simulink model "PID_Test"  (R2023b)
settings: Solver=VariableStepAuto  StartTime=0.0  StopTime=50  MaxStep=1  RelTol=1e-3  AbsTol=1e-3
InitFcn:
  | addpath('Schwungmasse/Schwungmasse_Matlab/Schwungmassenmodell_softHIL')
  | addpath('../');
  | 
  | if exist('systunePIDd', 'var')
  |     disp('systunePID exists!');
  | else
  |     MotorMitSchwungmasseTuner; % tune PID using systune
  | end
  | 
  | if ~exist('geneticPIDd', 'var') | ~exist('differentialPIDd', 'var')
  |     GeneticAndDifferentialParams; % init genetic and differential PIDs
  | end
undefined symbols (not defined in the file or in its folder): differentialPIDd, geneticPIDd, getservername, systunePIDd
libraries: slpidlib x3, simulink x2
settings Model: Creator=mkottman  LastModifiedBy=Alex
settings SolverCC: AutoScaleAbsTol=off  AlgebraicLoopSolver=TrustRegion
settings DataIOCC: SaveFormat=Array  SignalLoggingSaveFormat=ModelDataLogs  SaveOutput=off  SaveTime=off  ReturnWorkspaceOutputs=off
settings OptimizationCC: BooleanDataType=off  ExpressionDepthLimit=2147483647  InitFltsAndDblsToZero=on  LifeSpan=inf
settings DebuggingCC: SaveWithParameterizedLinksMsg=none  UnderspecifiedInitializationDetection=Classic  MergeDetectMultiDrivingBlocksExec=none  SignalResolutionControl=TryResolveAllWithWarning  MultiTaskDSMMsg=warning  MultiTaskCondExecSysMsg=none  FcnCallInpInsideContextMsg=warning  UnconnectedInputMsg=warning  UnconnectedOutputMsg=warning  UnconnectedLineMsg=warning  StateNameClashWarn=warning  SFUnexpectedBacktrackingDiag=warning  SFNoUnconditionalDefaultTransitionDiag=warning  SFExecutionAtInitializationDiag=none  ArithmeticOperatorsInVariantConditions=warning
settings HardwareCC: ProdBitPerPointer=32  ProdBitPerSizeT=32  ProdBitPerPtrDiffT=32  ProdLargestAtomicFloat=None  ProdIntDivRoundTo=Undefined  ProdEndianess=Unspecified  ProdWordSize=32  ProdHWDeviceType=32-bit Generic  TargetUnknown=on
settings ModelReferenceCC: EnableRefExpFcnMdlSchedulingChecks=on  PropagateSignalLabelsOutOfModel=off
settings SFSimCC: SimUseLocalCustomCode=off  CustomCodeUndefinedFunction=UseInterfaceOnly
settings RTWCC: TemplateMakefile=grt_vc.tmf  RTWUseLocalCustomCode=off
settings CodeAppCC: StateflowObjectComments=on
settings GRTTargetCC: TargetFcnLib=ansi_tfl_tmw.mat  TargetLangStandard=C89/C90 (ANSI)  CombineOutputUpdateFcns=off  GRTInterface=on
settings ConfigComp: CovMetricSettings=dw  CovSaveCumulativeToWorkspaceVar=on  CovSaveSingleToWorkspaceVar=on  CovExternalEMLEnable=off

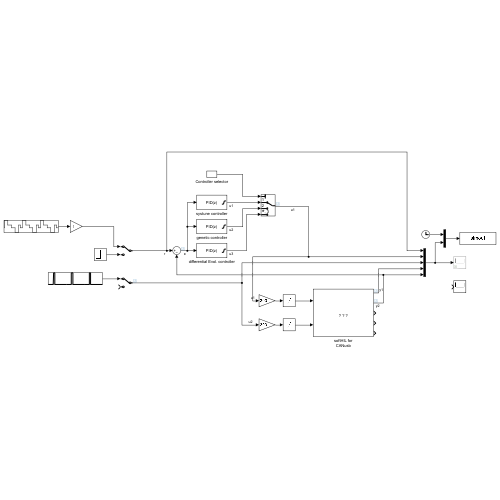
[thumbnail: Simulink's stored preview of the top-level diagram]
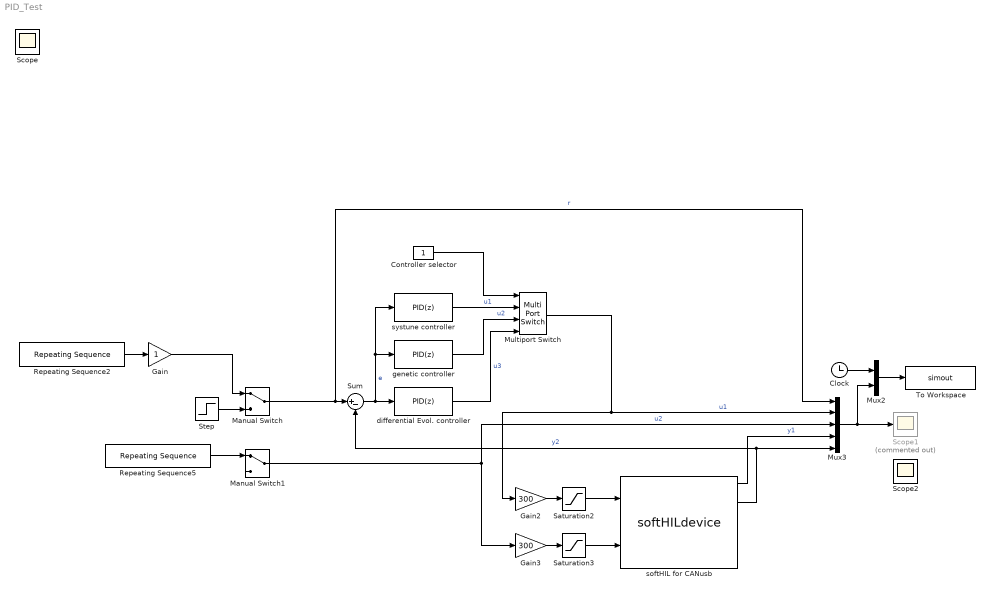
== system PID_Test ==
  Clock : Clock
  Controller selector : Constant
  Gain : Gain
  Gain2 : Gain  Gain=300
  Gain3 : Gain  Gain=300
  Manual Switch : ManualSwitch
  Manual Switch1 : ManualSwitch
  Multiport Switch : MultiPortSwitch  SaturateOnIntegerOverflow=off  InputSameDT=off
  Mux2 : Mux  Inputs=2
  Mux3 : Mux  Inputs=5
  Repeating Sequence2 : simulink/Sources/Repeating Sequence  rep_seq_t=[0.000000 0.490000 0.500000 9.990000 10.000000 19.990000 20.000000 29.990000 30.000000 39.990000 40.000000 44.990000 45.000000 49.990000 50.000000 ]  rep_seq_y=[0.000000 0.000000 31.415927 31.415927 12.566371 12.566371 0.000000 0.000000 -18.849556 -18.849556 12.566371 12.566371 0.000000 0.000000 0.000000 ]
  Repeating Sequence5 : simulink/Sources/Repeating Sequence  rep_seq_t=[0.000000 13.990000 14.000000 17.990000 18.000000 49.990000 50.000000 ]  rep_seq_y=[0.000000 0.000000 10.000000 10.000000 0.000000 0.000000 0.000000 ]
  Saturation2 : Saturate  UpperLimit=3000  LowerLimit=-3000
  Saturation3 : Saturate  UpperLimit=3000  LowerLimit=-3000
  Scope1 : Scope  Commented=on
  Scope2 : Scope
  Step : Step  Time=5  After=3.14159265/2  SampleTime=0.01
  Sum : Sum  Inputs=|+-
  To Workspace : ToWorkspace  VariableName=simout  SampleTime=0.01
  differential Evol. controller : slpidlib/PID Controller  Controller=PID  Form=Parallel  TimeDomain=Discrete-time  UseExternalTs=off  SampleTime=0.01  IntegratorMethod=Forward Euler  FilterMethod=Forward Euler  ControllerParametersSource=internal  P=differentialPIDd.Kp  I=differentialPIDd.Ki  UseKiTs=off  D=differentialPIDd.Kd  N=1/differentialPIDd.Tf  UseFilter=on  TunerSelectOption=Transfer Function Based (PID Tuner App)  InitialConditionSource=internal  InitialConditionForIntegrator=0  InitialConditionForFilter=0  DifferentiatorICPrevScaledInput=0  ExternalReset=none  TrackingMode=off  Kt=1  LimitOutput=on  SatLimitsSource=internal  UpperSaturationLimit=10  LowerSaturationLimit=-10  LinearizeAsGain=on  AntiWindupMode=clamping  Kb=1  LimitIntegrator=off  UpperIntegratorSaturationLimit=10  LowerIntegratorSaturationLimit=-10  POutMin=[]  POutMax=[]  IOutMin=[]  IOutMax=[]  DOutMin=[]  DOutMax=[]  NOutMin=[]  NOutMax=[]  SumOutMin=[]  SumOutMax=[]  SaturationOutMin=[]  SaturationOutMax=[]  PParamMin=[]  PParamMax=[]  IParamMin=[]  IParamMax=[]  DParamMin=[]  DParamMax=[]  NParamMin=[]  NParamMax=[]  KbParamMin=[]  KbParamMax=[]  KtParamMin=[]  KtParamMax=[]  KbOutMin=[]  KbOutMax=[]  KtOutMin=[]  KtOutMax=[]  IntegratorOutMin=[]  IntegratorOutMax=[]  FilterOutMin=[]  FilterOutMax=[]  SumI1OutMin=[]  SumI1OutMax=[]  SumI2OutMin=[]  SumI2OutMax=[]  SumI3OutMin=[]  SumI3OutMax=[]  SumI4OutMin=[]  SumI4OutMax=[]  SumDOutMin=[]  SumDOutMax=[]  DifferentiatorOutMin=[]  DifferentiatorOutMax=[]  FilterDiffOutCoefMin=[]  FilterDiffOutCoefMax=[]  ReciprocalOutMin=[]  ReciprocalOutMax=[]  SumDenOutMin=[]  SumDenOutMax=[]  SumNumOutMin=[]  SumNumOutMax=[]  DivideOutMin=[]  DivideOutMax=[]  UdiffTsProdOutMin=[]  UdiffTsProdOutMax=[]  NTsProdOutMin=[]  NTsProdOutMax=[]  UintegralTsProdOutMin=[]  UintegralTsProdOutMax=[]  UngainTsProdOutMin=[]  UngainTsProdOutMax=[]  ClampingZeroOutDataTypeStr=Inherit: Inherit via back propagation  ClampingZeroOutMin=[]  ClampingZeroOutMax=[]  FilterDenConstantOutDataTypeStr=Inherit: Inherit via back propagation  FilterDenConstantOutMin=[]  FilterDenConstantOutMax=[]  PCopyOutDataTypeStr=Inherit: Inherit via back propagation  PCopyOutMin=[]  PCopyOutMax=[]  NCopyOutDataTypeStr=Inherit: Inherit via back propagation  NCopyOutMin=[]  NCopyOutMax=[]  IntegratorContinuousStateAttributes=''  IntegratorStateMustResolveToSignalObject=off  IntegratorRTWStateStorageClass=Auto  FilterContinuousStateAttributes=''  FilterStateMustResolveToSignalObject=off  FilterRTWStateStorageClass=Auto  ParallelPVariant=InternalParameters  IdealPVariant=Disabled  IVariant=InternalParameters  DVariant=InternalParameters  IntegratorVariant=Discrete  SatVariant=Enabled  AWVariant=DiscClampingParallel  PCopyVariant=Disabled  TRVariant=Disabled  FdbkBlocksVariant=Forward  IdealPFdbkVariant=Disabled  SatFdbkVariant=Disabled  DerivativeFilterVariant=ForwardEulerFilter  NVariant=InternalParameters  NCopyVariant=Disabled  FilterICVariant=InternalICsFilter  IntegratorICVariant=InternalICs  ExternalResetVariant=Disabled  TRSumVariant=Passthrough  SumFdbkVariant=Disabled  SumVariant=Sum_PID  TsampFilterVariant=InternalTs  TsampNgainVariant=Passthrough  TsampIntegralVariant=Disabled_SignalSpec  ExternalSaturationOutDataTypeStr=Inherit: Same as second input
  genetic controller : slpidlib/PID Controller  Controller=PID  Form=Parallel  TimeDomain=Discrete-time  UseExternalTs=off  SampleTime=0.01  IntegratorMethod=Forward Euler  FilterMethod=Forward Euler  ControllerParametersSource=internal  P=geneticPIDd.Kp  I=geneticPIDd.Ki  UseKiTs=off  D=geneticPIDd.Kd  N=1/geneticPIDd.Tf  UseFilter=on  TunerSelectOption=Transfer Function Based (PID Tuner App)  InitialConditionSource=internal  InitialConditionForIntegrator=0  InitialConditionForFilter=0  DifferentiatorICPrevScaledInput=0  ExternalReset=none  TrackingMode=off  Kt=1  LimitOutput=on  SatLimitsSource=internal  UpperSaturationLimit=10  LowerSaturationLimit=-10  LinearizeAsGain=on  AntiWindupMode=clamping  Kb=1  LimitIntegrator=off  UpperIntegratorSaturationLimit=10  LowerIntegratorSaturationLimit=-10  POutMin=[]  POutMax=[]  IOutMin=[]  IOutMax=[]  DOutMin=[]  DOutMax=[]  NOutMin=[]  NOutMax=[]  SumOutMin=[]  SumOutMax=[]  SaturationOutMin=[]  SaturationOutMax=[]  PParamMin=[]  PParamMax=[]  IParamMin=[]  IParamMax=[]  DParamMin=[]  DParamMax=[]  NParamMin=[]  NParamMax=[]  KbParamMin=[]  KbParamMax=[]  KtParamMin=[]  KtParamMax=[]  KbOutMin=[]  KbOutMax=[]  KtOutMin=[]  KtOutMax=[]  IntegratorOutMin=[]  IntegratorOutMax=[]  FilterOutMin=[]  FilterOutMax=[]  SumI1OutMin=[]  SumI1OutMax=[]  SumI2OutMin=[]  SumI2OutMax=[]  SumI3OutMin=[]  SumI3OutMax=[]  SumI4OutMin=[]  SumI4OutMax=[]  SumDOutMin=[]  SumDOutMax=[]  DifferentiatorOutMin=[]  DifferentiatorOutMax=[]  FilterDiffOutCoefMin=[]  FilterDiffOutCoefMax=[]  ReciprocalOutMin=[]  ReciprocalOutMax=[]  SumDenOutMin=[]  SumDenOutMax=[]  SumNumOutMin=[]  SumNumOutMax=[]  DivideOutMin=[]  DivideOutMax=[]  UdiffTsProdOutMin=[]  UdiffTsProdOutMax=[]  NTsProdOutMin=[]  NTsProdOutMax=[]  UintegralTsProdOutMin=[]  UintegralTsProdOutMax=[]  UngainTsProdOutMin=[]  UngainTsProdOutMax=[]  ClampingZeroOutDataTypeStr=Inherit: Inherit via back propagation  ClampingZeroOutMin=[]  ClampingZeroOutMax=[]  FilterDenConstantOutDataTypeStr=Inherit: Inherit via back propagation  FilterDenConstantOutMin=[]  FilterDenConstantOutMax=[]  PCopyOutDataTypeStr=Inherit: Inherit via back propagation  PCopyOutMin=[]  PCopyOutMax=[]  NCopyOutDataTypeStr=Inherit: Inherit via back propagation  NCopyOutMin=[]  NCopyOutMax=[]  IntegratorContinuousStateAttributes=''  IntegratorStateMustResolveToSignalObject=off  IntegratorRTWStateStorageClass=Auto  FilterContinuousStateAttributes=''  FilterStateMustResolveToSignalObject=off  FilterRTWStateStorageClass=Auto  ParallelPVariant=InternalParameters  IdealPVariant=Disabled  IVariant=InternalParameters  DVariant=InternalParameters  IntegratorVariant=Discrete  SatVariant=Enabled  AWVariant=DiscClampingParallel  PCopyVariant=Disabled  TRVariant=Disabled  FdbkBlocksVariant=Forward  IdealPFdbkVariant=Disabled  SatFdbkVariant=Disabled  DerivativeFilterVariant=ForwardEulerFilter  NVariant=InternalParameters  NCopyVariant=Disabled  FilterICVariant=InternalICsFilter  IntegratorICVariant=InternalICs  ExternalResetVariant=Disabled  TRSumVariant=Passthrough  SumFdbkVariant=Disabled  SumVariant=Sum_PID  TsampFilterVariant=InternalTs  TsampNgainVariant=Passthrough  TsampIntegralVariant=Disabled_SignalSpec  ExternalSaturationOutDataTypeStr=Inherit: Same as second input
  softHIL for CANusb : S-Function  FunctionName=softHILdevice  Parameters=nAIn, nAOut, nDIn, nDOut, 0, Sampletime, Servername, ServerOL, ClientOL, Delay, 'CANusb'  SFunctionDeploymentMode=off  EnableBusSupport=off  mask(softHIL for the CANusb){nAIn=2, nAOut=2, nDIn=0, nDOut=0, Sampletime=0.01, Servername=getservername, ServerOL=on, ClientOL=on, Delay=on}
      mask prompts: nAIn "Number of Analog In (AI)"; nAOut "Number of Analog Out (AO)"; nDIn "Number of Digital In (DI)"; nDOut "Number of Digital Out (DO)"; Sampletime "Sample Time"; ServerOL "Show Server Overloads Port"; ClientOL "Show Client Overloads Port"; Delay "Show Roundtrip Delay Port"
      mask help: softHIL (soft hardware in the loop) for the CANusb device.
      mask Help:
      | softHIL (soft hardware in the loop) for the CANusb allows to connect to a remote server (over TCP and UDP) which runs the SoftHILServer service to acquire from and deliver data to the device. This version is limited to work for the setup at the Control Engineering Laboratories of the University of Applied Sciences HSR in Rapperswil, CH.
      | 
      | The implementation of the softing CANusb device was only made for the process “Schwungmasse“. If you want to use the device in a different function it’s recommended to use it directly.
      | 
      | <big><b>Ports</b></big>
      | <table border=1><tr><td>Portname</td><td>Description</td><td>Min</td><td>Max</td></tr><tr><td>AO1/A2</td><td>Analog Outputs</td><td>-</td><td>-</td></tr><tr><td>AI1/AI2</td><td>Analog Inputs</td><td>-</td><td>-</td></tr><tr><td>SOL</td><td>Whenever the server is not able to finish the acquisition of the samples at the specified sample time, a server overload occurs and the SOL (Server Overloads) counter will increment by 1.</td><td>0</td><td>2^31</td></tr><tr><td>COL</td><td>Whenever the client is not able to finish its calculations until the next samples arrive, a client overload occurs and the COL (Client Overloads) counter will increment by 1.</td><td>0</td><td>2^31</td></tr><tr><td>tau</td><td>tau specifies the current roundtrip delay. It is a measure of the delay due to the network (protocol stack, switches, etc.)</td><td>0</td><td>-</td></tr></table>
      | <br>
      | <big><b>Parameters</b></big>
      | <table border="1"><tr><td>Parametername</td><td>Description</td><td>Min</td><td>Max</td></tr><tr><td>Number of Analog In (AI)</td><td>A scalar value that specifies the number of analog input channels the I/O board should acquire. Should be 2!</td><td>0</td><td>8</td></tr><tr><td>Number of Analog Out (AO)</td><td>A scalar value that specifies the number of analog output channels the I/O board should write to. Should be 2!</td><td>0</td><td>6</td></tr><tr><td>Number of Digital In (DI)</td><td>A scalar value that specifies the number of digital input channels the I/O board should acquire. Should be 0!</td><td>0</td><td>8</td></tr><tr><td>Number of Digital Out (DO)</td><td>A scalar value that specifies the number of digital output channels the I/O board should set. Should be 0!</td><td>0</td><td>8</td></tr><tr><td>Sample Time</td><td>A scalar value that specifies the sampling rate (in seconds) at which the I/O board acquires data and at which rate the softHIL block sends new output values to the server. The rate has to be a multiple of 1ms.</td><td>0.001</td><td>-</td></tr><tr><td>Servername</td><td>The name or IP address of the server on which the SoftHILServer service is running and the I/O boards are installed. This argument has to be a string. Use 'localhost' if the server runs on the same machine.</td><td>-</td><td>-</td></tr><tr><td>Show Server Overload Port</td><td>Check to see the 'SOL' output port.</td><td>-</td><td>-</td></tr><tr><td>Show Client Overload Port</td><td>Check to see the 'COL' output port.</td><td>-</td><td>-</td></tr><tr><td>Show Roundtrip Delay Port</td><td>Check to see the 'tau' output port.</td><td>-</td><td>-</td></tr></table>
      | <br>
      | <big style="font-weight: bold;">Hints</big><br>
      | <ul>
      | <li>It can happen that Simulink freezes during simulation due to a connection problem with the server. In this case, restart the SoftHILServer service on the server. As soon as the service quits, Simulink will enter a normal error state and stop the simulation. Check the Event Log of the server to get some information about the cause of the problem.</li>
      | <li>When you receive a 'configuration error' and the Simulation does not start, make sure that the number of channels are in the correct range and check the Event Log on the server for further information. Make sure to have the correct InstaCal installed on the server and the boards are properly configured.</li>
      | <li>The server and the client run on Windows, which is not a RealTime operating system. Execution accuracy depends on the available system resources. Do not do anything else with the system during simulations to improve accuracy.</li>
      | <li>Check SOL and COL output ports to make sure the server and the client are able to deliver the required sample time. Some overloads during the start of the simulation are normal. While the simulation is running, these counters should not continuously increase. If this happens, the RealTime condition is hardly violated. Increase the sample time and/or reduce model complexity.</li>
      | <li>The more values are read from and written to the I/O board, the longer the A/D and D/A conversions will take. It is possible that the lower bound of 1ms is not possible any more, even for the simplest model and fastes processors. Check the server overload counter (SOL) to detect this problem.</li>
      | </ul>
      mask Display:
      | image(imread('CANusb.jpg'));
      | 
      | nAIn = str2num(get_param(gcb, 'nAIn'));
      | nDIn = str2num(get_param(gcb, 'nDIn'));
      | nAOut = str2num(get_param(gcb, 'nAOut'));
      | nDOut = str2num(get_param(gcb, 'nDOut'));
      | 
      | offset = 0;
      | for i = 1:nAIn
      |     port_label('output', i + offset, ['AI' num2str(i)]);
      | end
      | offset = offset + nAIn;
      | for i = 1:nDIn
      |     port_label('output', i + offset, ['DI', num2str(i)]);
      | end
      | offset = offset + nDIn;
      | if strcmp(get_param(gcb, 'ServerOL'), 'on')
      |     port_label('output', 1 + offset, 'SOL');
      |     offset = offset + 1;
      | end
      | if strcmp(get_param(gcb, 'ClientOL'), 'on')
      |     port_label('output', 1 + offset, 'COL');
      |     offset = offset + 1;
      | end
      | if strcmp(get_param(gcb, 'Delay'), 'on')
      |     port_label('output', 1 + offset, 'tau');
      |     offset = offset + 1;
      | end
      | 
      | offset = 0;
      | for i = 1:nAOut
      |     port_label('input', i + offset, ['AO' num2str(i)]);
      | end
      | offset = offset + nAOut;
      | for i = 1:nDOut
      |     port_label('input', i + offset, ['DO', num2str(i)]);
      | end
  systune controller : slpidlib/PID Controller  Controller=PID  Form=Parallel  TimeDomain=Discrete-time  UseExternalTs=off  SampleTime=0.01  IntegratorMethod=Forward Euler  FilterMethod=Forward Euler  ControllerParametersSource=internal  P=systunePIDd.Kp  I=systunePIDd.Ki  UseKiTs=off  D=systunePIDd.Kd  N=1/systunePIDd.Tf  UseFilter=on  TunerSelectOption=Transfer Function Based (PID Tuner App)  InitialConditionSource=internal  InitialConditionForIntegrator=0  InitialConditionForFilter=0  DifferentiatorICPrevScaledInput=0  ExternalReset=none  TrackingMode=off  Kt=1  LimitOutput=on  SatLimitsSource=internal  UpperSaturationLimit=10  LowerSaturationLimit=-10  LinearizeAsGain=on  AntiWindupMode=clamping  Kb=1  LimitIntegrator=off  UpperIntegratorSaturationLimit=10  LowerIntegratorSaturationLimit=-10  POutMin=[]  POutMax=[]  IOutMin=[]  IOutMax=[]  DOutMin=[]  DOutMax=[]  NOutMin=[]  NOutMax=[]  SumOutMin=[]  SumOutMax=[]  SaturationOutMin=[]  SaturationOutMax=[]  PParamMin=[]  PParamMax=[]  IParamMin=[]  IParamMax=[]  DParamMin=[]  DParamMax=[]  NParamMin=[]  NParamMax=[]  KbParamMin=[]  KbParamMax=[]  KtParamMin=[]  KtParamMax=[]  KbOutMin=[]  KbOutMax=[]  KtOutMin=[]  KtOutMax=[]  IntegratorOutMin=[]  IntegratorOutMax=[]  FilterOutMin=[]  FilterOutMax=[]  SumI1OutMin=[]  SumI1OutMax=[]  SumI2OutMin=[]  SumI2OutMax=[]  SumI3OutMin=[]  SumI3OutMax=[]  SumI4OutMin=[]  SumI4OutMax=[]  SumDOutMin=[]  SumDOutMax=[]  DifferentiatorOutMin=[]  DifferentiatorOutMax=[]  FilterDiffOutCoefMin=[]  FilterDiffOutCoefMax=[]  ReciprocalOutMin=[]  ReciprocalOutMax=[]  SumDenOutMin=[]  SumDenOutMax=[]  SumNumOutMin=[]  SumNumOutMax=[]  DivideOutMin=[]  DivideOutMax=[]  UdiffTsProdOutMin=[]  UdiffTsProdOutMax=[]  NTsProdOutMin=[]  NTsProdOutMax=[]  UintegralTsProdOutMin=[]  UintegralTsProdOutMax=[]  UngainTsProdOutMin=[]  UngainTsProdOutMax=[]  ClampingZeroOutDataTypeStr=Inherit: Inherit via back propagation  ClampingZeroOutMin=[]  ClampingZeroOutMax=[]  FilterDenConstantOutDataTypeStr=Inherit: Inherit via back propagation  FilterDenConstantOutMin=[]  FilterDenConstantOutMax=[]  PCopyOutDataTypeStr=Inherit: Inherit via back propagation  PCopyOutMin=[]  PCopyOutMax=[]  NCopyOutDataTypeStr=Inherit: Inherit via back propagation  NCopyOutMin=[]  NCopyOutMax=[]  IntegratorContinuousStateAttributes=''  IntegratorStateMustResolveToSignalObject=off  IntegratorRTWStateStorageClass=Auto  FilterContinuousStateAttributes=''  FilterStateMustResolveToSignalObject=off  FilterRTWStateStorageClass=Auto  ParallelPVariant=InternalParameters  IdealPVariant=Disabled  IVariant=InternalParameters  DVariant=InternalParameters  IntegratorVariant=Discrete  SatVariant=Enabled  AWVariant=DiscClampingParallel  PCopyVariant=Disabled  TRVariant=Disabled  FdbkBlocksVariant=Forward  IdealPFdbkVariant=Disabled  SatFdbkVariant=Disabled  DerivativeFilterVariant=ForwardEulerFilter  NVariant=InternalParameters  NCopyVariant=Disabled  FilterICVariant=InternalICsFilter  IntegratorICVariant=InternalICs  ExternalResetVariant=Disabled  TRSumVariant=Passthrough  SumFdbkVariant=Disabled  SumVariant=Sum_PID  TsampFilterVariant=InternalTs  TsampNgainVariant=Passthrough  TsampIntegralVariant=Disabled_SignalSpec  ExternalSaturationOutDataTypeStr=Inherit: Same as second input
  Scope : Scope
  wires:
  Step/1 -> Manual Switch/2
  Sum/1 -> systune controller/1, genetic controller/1, differential Evol. controller/1  "e"
  Manual Switch/1 -> Mux3/1, Sum/1  "r"
  Repeating Sequence2/1 -> Gain/1
  softHIL for CANusb/2 -> Sum/2, Mux3/5  "y2"
  softHIL for CANusb/1 -> Mux3/4  "y1"
  Mux3/1 -> Scope1/1, Mux2/2
  Manual Switch1/1 -> Gain3/1, Mux3/3  "u2"
  Repeating Sequence5/1 -> Manual Switch1/1
  Mux2/1 -> To Workspace/1
  Clock/1 -> Mux2/1
  Gain/1 -> Manual Switch/1
  Multiport Switch/1 -> Mux3/2, Gain2/1  "u1"
  Controller selector/1 -> Multiport Switch/1
  systune controller/1 -> Multiport Switch/2  "u1"
  genetic controller/1 -> Multiport Switch/3  "u2"
  differential Evol. controller/1 -> Multiport Switch/4  "u3"
  Gain2/1 -> Saturation2/1
  Saturation2/1 -> softHIL for CANusb/1
  Gain3/1 -> Saturation3/1
  Saturation3/1 -> softHIL for CANusb/2
